simulink model "MoboticPositionFeedback_DataCast"  (R2024a)
settings: Solver=VariableStepAuto  StartTime=0.0  StopTime=10.0  RelTol=1e-3
settings Model: Creator=ander  LastModifiedBy=ander

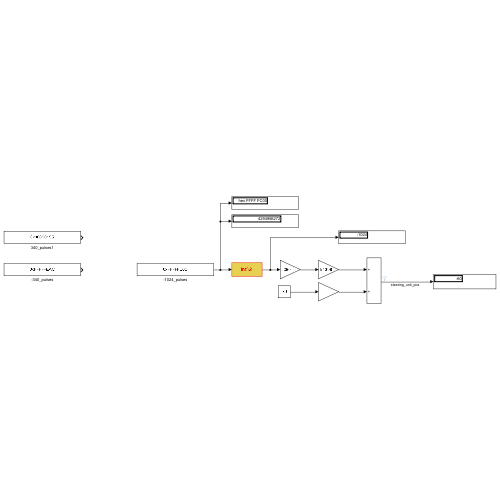
[thumbnail: Simulink's stored preview of the top-level diagram]
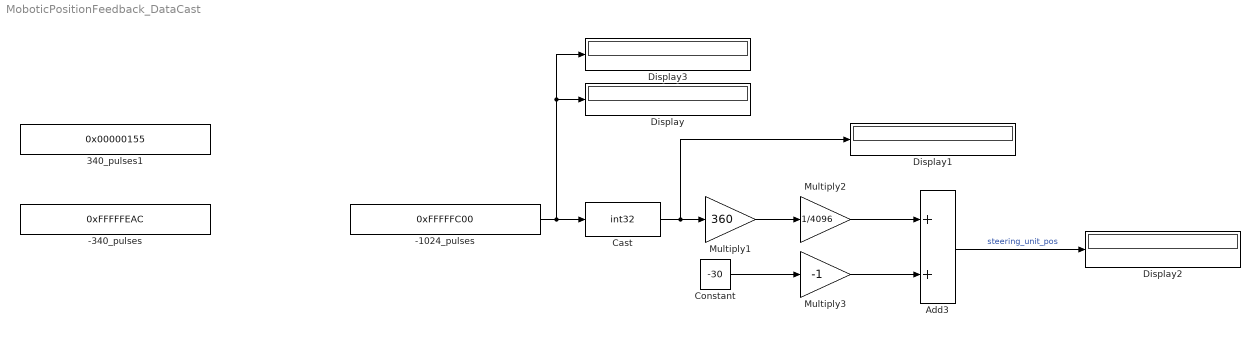
== system MoboticPositionFeedback_DataCast ==
  -1024_pulses : Constant  Value=0xFFFFFC00
  -340_pulses : Constant  Value=0xFFFFFEAC
  340_pulses1 : Constant  Value=0x00000155
  Add3 : Sum
  Cast : DataTypeConversion  OutDataTypeStr=int32  SaturateOnIntegerOverflow=off  RndMeth=Floor
  Constant : Constant  Value=-30
  Display{,1..3} (4 alike) : Display
      Display3 settings: Format=hex (Stored Integer)
  Multiply1 : Gain  Gain=360
  Multiply2 : Gain  Gain=1/4096
  Multiply3 : Gain  Gain=-1
  wires:
  Multiply3/1 -> Add3/2
  Multiply1/1 -> Multiply2/1
  Multiply2/1 -> Add3/1
  Constant/1 -> Multiply3/1
  Cast/1 -> Display1/1, Multiply1/1
  -1024_pulses/1 -> Display3/1, Display/1, Cast/1
  Add3/1 -> Display2/1  "steering_unit_pos"
